simulink subsystem "EncoderAdrydis"  (R2023b)
settings: Solver=VariableStepAuto  StartTime=0.0  StopTime=10.0  RelTol=1e-3
libraries: arduinosensorlib x2
settings Model: Creator=johan  LastModifiedBy=adria

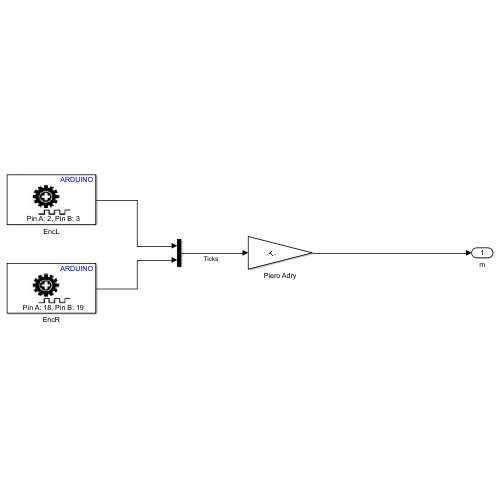
[thumbnail: Simulink's stored preview of the top-level diagram]
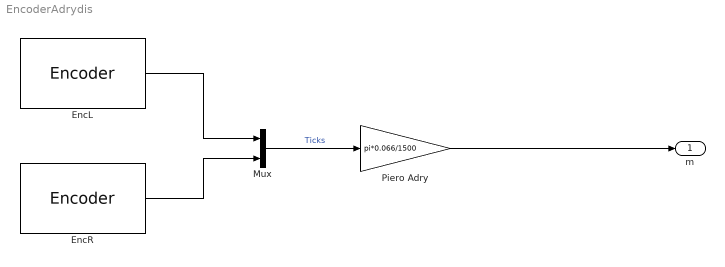
== system EncoderAdrydis ==
  EncL : arduinosensorlib/Encoder  InputA=2  InputB=3  Mode=No reset  SampleTime=-1
  EncR : arduinosensorlib/Encoder  InputA=18  InputB=19  Mode=No reset  SampleTime=-1
  Mux : Mux  Inputs=2
  Piero Adry : Gain  Gain=pi*0.066/1500
  m : Outport
  wires:
  Piero Adry/1 -> m/1
  Mux/1 -> Piero Adry/1  "Ticks"
  EncR/1 -> Mux/2
  EncL/1 -> Mux/1
